simulink model "AutoFollow_Simulation"  (R2014a)
settings: Solver=ode45  StartTime=0.0  StopTime=50  FixedStep=0.05  MaxStep=0.06  RelTol=1e-3
model workspace (MAT data in the model file):
  MCOS : class17 (value not decoded)
undefined symbols (not defined in the file or in its folder): IC, quadModel
libraries: simulink x4, commnoisgen2 x2
(part 2 of 2)

== matlab function AutoFollow_Simulation/Kalman Filter/MATLAB Function ==
  settings: updateMethod=DISCRETE  sampleTime=0.02
  data: hx_cam input; hy_cam input; hz_cam input; u input; v input; w input; newMeas input; t input; xhatOut output
function xhatOut = kalman(hx_cam, hy_cam, hz_cam, u, v, w, newMeas, t)
% http://www.goddardconsulting.ca/simulink-extended-kalman-filter-tracking.html
% http://www.physicspages.com/2012/12/24/coordinate-transformations-the-jacobian-determinant/
% The states of the process are given by
% x = [x_position; y_position; z_position; x_velocity; y_velocity; z_velocity];
%
% and the measurements are given by
% y = [x_position; y_position; z_position]

persistent prevT prevY P xhat Q R
%% First time through the code so do some initialization
if isempty(P)
   %initial state estimate
   xhat = [0;0;10;0;0;0];
   
   % current state varience
   P = zeros(6,6);
   
   % covarience matrix for state propagation
   Q = diag([10 10 40 400 400 1400].^2);
   
   % covarience matrix for sensor updates
   R = diag([5 5 200].^2);
   
   % last time step
   prevT = 0;
   
   % previous sensor measurements
   prevY = [0;0;0];
end
dt = t - prevT;

%% State space matricies
velSlowDown = 8;
A = [1 0 0 dt/velSlowDown 0 0;
     0 1 0 0 dt/velSlowDown 0;
     0 0 1 0 0 dt/velSlowDown;
     0 0 0 1 0 0;
     0 0 0 0 1 0;
     0 0 0 0 0 1];
 
u = [u;v;w];
B = [-1 0 0;
     0 -1 0;
     0 0 -1;
     0 0 0;
     0 0 0;
     0 0 0];

C = [1 0 0 0 0 0;
     0 1 0 0 0 0;
     0 0 1 0 0 0];
 
%% predictor step
xhat = A*xhat;% + B*u;
% xhat(1) = xhat(1) - u*dt;
% xhat(2) = xhat(2) - v*dt;
% xhat(3) = xhat(3) - w*dt;
P = A*P*A' + Q;

%% corrector step
y = [hx_cam; hy_cam; hz_cam];

% if newMeas
if (abs(y(1) - prevY(1)) > 0.02 && ...
    abs(y(2) - prevY(2)) > 0.02 && ...
    abs(y(3) - prevY(3)) > 0.02) && ...
    newMeas
    fprintf('time: %f, hx: %f, hy: %f\n', t, hx_cam, hy_cam);
    K = P*C'/(C*P*C' + R);
    xhat = xhat + K*(y - C*xhat);
    P = (eye(size(K,1)) - K*C)*P;
    prevY = y;
end


%% results
xhatOut = xhat;

end

== matlab function AutoFollow_Simulation/Kalman Filter/MATLAB Function1 ==
  settings: updateMethod=DISCRETE  sampleTime=0.02
  data: thetaq input; hx output; psiq input; phiq input; hr input; htheta input; hpsi input; hy output; hz output
function [hx, hy, hz] = cam2global(thetaq, psiq, phiq, hr, htheta, hpsi)
% camera coordinates to global 
%transform r, theta, psi to x, y, z
[hx, hy, hz] = sphere2cart(hr, htheta, hpsi);
%rotate into global frame
Rback = [cos(psiq)*cos(thetaq) cos(psiq)*sin(thetaq)*sin(phiq)-sin(psiq)*cos(phiq) cos(psiq)*sin(thetaq)*cos(phiq)+sin(psiq)*sin(phiq);
          sin(psiq)*cos(thetaq) sin(psiq)*sin(thetaq)*sin(phiq)+cos(psiq)*cos(phiq) sin(psiq)*sin(thetaq)*cos(phiq)-cos(psiq)*sin(phiq);
          -sin(thetaq)         cos(thetaq)*sin(phiq)                            cos(thetaq)*cos(phiq)];
cam = [hx; hy; hz];
human = Rback*cam;

hx = human(1);
hy = human(2);
hz = human(3);
end

function [x, y, z] = sphere2cart(r, theta, psi)
x = r.*sin(psi).*cos(theta);
y = r.*sin(psi).*sin(theta);
z = r.*cos(psi);
end

== matlab function AutoFollow_Simulation/Kalman Filter/MATLAB Function2 ==
  settings: updateMethod=DISCRETE  sampleTime=0.02
  data: thetaq input; phiq input; psiq input; hr input; htheta input; hpsi input; xhatOut output; t input
function xhatOut = EKF(thetaq, phiq, psiq, hr, htheta, hpsi, t)
% http://www.goddardconsulting.ca/simulink-extended-kalman-filter-tracking.html
% http://www.physicspages.com/2012/12/24/coordinate-transformations-the-jacobian-determinant/
% The states of the process are given by
% x = [x_position; y_position; z_position; x_velocity; y_velocity; z_velocity];
%
% and the measurements are given by
% y = [r; theta; psi]

persistent prevT prevMeas P xhat Q R
%% First time through the code so do some initialization
if isempty(P)
   %initial state estimate
   xhat = [0;0;-10;0;0;0];
   
   % current state varience
   P = zeros(6,6);
   
   % covarience matrix for state propagation
   Q = diag([0 0 0 .1 .1 .1]);
   
   % covarience matrix for sensor updates
   R = diag([5^2 5^2 50^2]);
   
   % last time step
   prevT = 0;
   
   % previous sensor measurements
   prevMeas = [0;0;0];
end
dt = t - prevT;

%% A matrix
A = [1 0 0 dt 0 0;
     0 1 0 0 dt 0;
     0 0 1 0 0 dt;
     0 0 0 1 0 0;
     0 0 0 0 1 0;
     0 0 0 0 0 1];
%% setup for C matrix
cart = [hr*sin(hpsi)*cos(htheta); 
        hr*sin(hpsi)*sin(htheta);
        hr*cos(hpsi)];

R = [cos(psiq)*cos(thetaq) cos(psiq)*sin(thetaq)*sin(phiq)-sin(psiq)*cos(phiq) cos(psiq)*sin(thetaq)*cos(phiq)+sin(psiq)*sin(phiq);
     sin(psiq)*cos(thetaq) sin(psiq)*sin(thetaq)*sin(phiq)+cos(psiq)*cos(phiq) sin(psiq)*sin(thetaq)*cos(phiq)-cos(psiq)*sin(phiq);
     -sin(thetaq)         cos(thetaq)*sin(phiq)                            cos(thetaq)*cos(phiq)];
cart = R*cart;
x = cart(1);
y = cart(2);
z = cart(3);
r = sqrt(x^2 + y^2 + z^2);
theta = atan2(y, z);
psi = atan2(sqrt(x^2+y^2),z);

dr_dx = x/r;
dr_dy = y/r;
dr_dz = z/r;
dtheta_dx = x*z/(r^3 * sin(theta));
dtheta_dy = y*z/(r^3 * sin(theta));
dtheta_dz = -sin(theta)/r;
dpsi_dx = -y/(r^2 * sin(theta)^2);
dpsi_dy = x/(r^2 * sin(theta)^2);
dpsi_dz = 0;

%all partials of velocity are 0;
    % dx, dy, dz, dvx, dvy, dvz
C = [dr_dx     dr_dy     dr_dz     0 0 0;
     dtheta_dx dtheta_dy dtheta_dz 0 0 0;
     dpsi_dx   dpsi_dy   dpsi_dz   0 0 0];
 
%% predictor step
xhat = A*xhat;
P = A*P*A' + Q;

%% corrector step
meas = [r; theta; psi];

if (meas(1) == prevMeas(1)) && (meas(2) == prevMeas(2)) && (meas(3) == prevMeas(3))
    K = P*C'/(C*P*C' + R);
    xhat = xhat + K*(meas - C*xhat);
    P = (eye(size(K,1)) - K*C)*P;
end
prevMeas = meas;

%% results
xhatOut = xhat;

end
